simulink model "gm_HDLAWGNGenerator"  (R2021a)
settings: Solver=FixedStepDiscrete  StartTime=0.0  StopTime=StopTime  RelTol=1e-3
InitFcn:
  | whdlexamples.hdlawgn_init
undefined symbols (not defined in the file or in its folder): coefficientsSqrt1, coefficientsSqrt2, SamplingTime, seedsURNG1, seedsURNG2
libraries: hdlsllib x22, simulink x21, dspsrcs4 x1
(part 1 of 2)
settings Model: SimulationMode=accelerator  Creator=The MathWorks, Inc.  LastModifiedBy=huber
settings SolverCC: AlgebraicLoopSolver=TrustRegion
settings DataIOCC: ReturnWorkspaceOutputs=off
settings OptimizationCC: BlockReduction=off  ConditionallyExecuteInputs=off  DefaultParameterBehavior=Inlined
settings DebuggingCC: AlgebraicLoopMsg=error  InheritedTsInSrcMsg=none  SingleTaskRateTransMsg=error  IntegerOverflowMsg=none  ParameterPrecisionLossMsg=none  SFMachineParentedDataDiag=warning
settings HardwareCC: ProdBitPerPointer=32  ProdBitPerSizeT=32  ProdBitPerPtrDiffT=32  ProdLargestAtomicFloat=None  ProdIntDivRoundTo=Undefined  ProdEndianess=Unspecified  ProdWordSize=32  ProdHWDeviceType=ASIC/FPGA->ASIC/FPGA  TargetBitPerPointer=64  TargetBitPerSizeT=64  TargetBitPerPtrDiffT=64  TargetLongLongMode=on  TargetIntDivRoundTo=Zero  TargetEndianess=LittleEndian  TargetWordSize=64  TargetHWDeviceType=Custom Processor->MATLAB Host Computer  ProdEqTarget=off

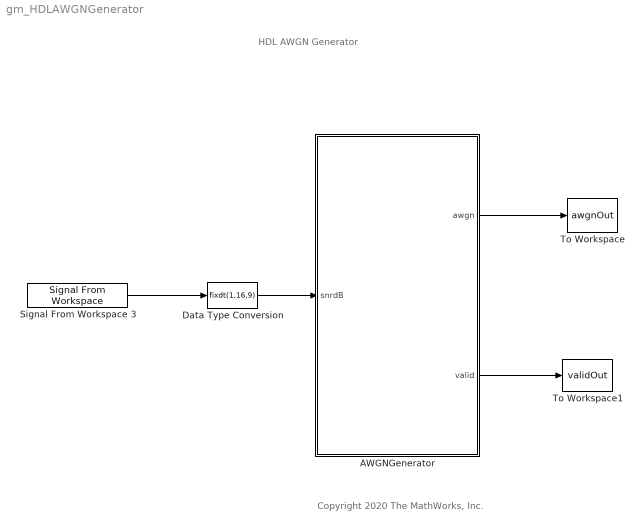
== system gm_HDLAWGNGenerator ==
  note: Copyright 2020 The MathWorks, Inc.
  note: HDL AWGN Generator
  AWGNGenerator : Subsystem
  Data Type Conversion : DataTypeConversion  OutDataTypeStr=fixdt(1,16,9)
  Signal From Workspace 3 : dspsrcs4/Signal From Workspace  X=snrdBSimInput  Ts=SamplingTime  nsamps=1  OutputAfterFinalValue=Setting to zero  ignoreOrWarnInputAndFrameLengths=on  OutputFrames=off
  To Workspace : ToWorkspace  VariableName=awgnOut  SampleTime=-1
      settings: Save2DSignal=2-D array (concatenate along first dimension)
  To Workspace1 : ToWorkspace  VariableName=validOut  SampleTime=-1
      settings: Save2DSignal=2-D array (concatenate along first dimension)
  wires:
  AWGNGenerator/2(valid) -> To Workspace1/1
  AWGNGenerator/1(awgn) -> To Workspace/1
  Data Type Conversion/1 -> AWGNGenerator/1(snrdB)
  Signal From Workspace 3/1 -> Data Type Conversion/1

== system gm_HDLAWGNGenerator/AWGNGenerator ==
  snrdB : Inport  OutDataTypeStr=fixdt(1, 16, 9)  PortDimensions=1  SampleTime=1e-06
  " dBtoLinearConverter" : Subsystem
  Data Type Conversion1 : DataTypeConversion  OutDataTypeStr=fixdt(1,16,9)
  Delay1 : Delay  DelayLength=10
  GaussianNoiseWithReqVar : Subsystem
  GaussianNoiseWithUnitVar : Subsystem
  awgn : Outport  SampleTime=1e-06
  valid : Outport  Port=2  SampleTime=1e-06
  wires:
  snrdB/1 -> Data Type Conversion1/1
  " dBtoLinearConverter"/1(noiseVar) -> Delay1/1
  Data Type Conversion1/1 -> " dBtoLinearConverter"/1(snrdB)
  Delay1/1 -> GaussianNoiseWithReqVar/1(noiseVar)
  GaussianNoiseWithReqVar/1(awgn) -> awgn/1
  GaussianNoiseWithReqVar/2(validOut) -> valid/1
  GaussianNoiseWithUnitVar/1(x0) -> GaussianNoiseWithReqVar/2(x0)
  GaussianNoiseWithUnitVar/2(x1) -> GaussianNoiseWithReqVar/3(x1)

== system gm_HDLAWGNGenerator/AWGNGenerator/ dBtoLinearConverter ==
  snrdB : Inport  OutDataTypeStr=fixdt(1, 16, 9)  PortDimensions=1  SampleTime=1e-06
  Add : Sum  AccumDataTypeStr=int16  OutDataTypeStr=int16  SampleTime=1e-06
  Constant : Constant  Value=201  OutDataTypeStr=int16  SampleTime=1e-06
  Delay1 : Delay  DelayLength=double(1)  InitialCondition=0  SampleTime=1e-06
  Gain : Gain  Gain="fi(0,1,16,11,\"hex\",\"5000\")"  ParamDataTypeStr=fixdt(1, 16, 11)  OutDataTypeStr=fixdt(1, 32, 20)  SampleTime=1e-06
  Gain_out_dtc : DataTypeConversion  OutDataTypeStr=int16  RndMeth=Round  SampleTime=1e-06
  sqrt(noisePow/2) : Lookup_n-D  NumberOfTableDimensions=1  BreakpointsForDimension1="fi(\"numerictype\",numerictype(1,16,0),\"fimath\",fimath(\"RoundingMethod\", \"Nearest\",\"OverflowAction\", \"Saturate\",\"ProductMode\",\"FullPrecision\",\"SumMode\",\"FullPrecision\"),\"Value\",\"[0 1 2 3 4 5 6 7 8 9 10 11 12 13 14 15 16 17 18 19 20 21 22 23 24 25 26 27 28 29 30 31 32 33 34 35 36 37 38 39 40 41 42 43 44 45 46 47 48 49 50 51 52 53 54 55 56 57 58 59 60 61 62 63 64 65 66 67 68 69 70 71 72 73 74 75 76 77 78 79 80 81 82 83 84 85 86 87 88 89 90 91 92 93 94 95 96 97 98 99 100 101 102 103 104 105 106 107 108 109 110 111 112 113 114 115 116 117 118 119 120 121 122 123 124 125 126 127 128 129 130 131 132 133 134 135 136 137 138 139 140 141 142 143 144 145 146 147 148 149 150 151 152 153 154 155 156 157 158 159 160 161 162 163 164 165 166 167 168 169 170 171 172 173 174 175 176 177 178 179 180 181 182 183 184 185 186 187 188 189 190 191 192 193 194 195 196 197 198 199 200 201 202 203 204 205 206 207 208 209 210 211 212 213 214 215 216 217 218 219 220 221 222 223 224 225 226 227 228 229 230 231 232 233 234 235 236 237 238 239 240 241 242 243 244 245 246 247 248 249 250 251 252 253 254 255 256 257 258 259 260 261 262 263 264 265 266 267 268 269 270 271 272 273 274 275 276 277 278 279 280 281 282 283 284 285 286 287 288 289 290 291 292 293 294 295 296 297 298 299 300 301 302 303 304 305 306 307 308 309 310 311 312 313 314 315 316 317 318 319 320 321 322 323 324 325 326 327 328 329 330 331 332 333 334 335 336 337 338 339 340 341 342 343 344 345 346 347 348 349 350 351 352 353 354 355 356 357 358 359 360 361 362 363 364 365 366 367 368 369 370 371 372 373 374 375 376 377 378 379 380 381 382 383 384 385 386 387 388 389 390 391 392 393 394 395 396 397 398 399 400 401 402 403 404 405 406 407 408 409 410 411 412 413 414 415 416 417 418 419 420 421 422 423 424 425 426 427 428 429 430 431 432 433 434 435 436 437 438 439 440 441 442 443 444 445 446 447 448 449 450 451 452 453 454 455 456 457 458 459 460 461 462 463 464 465 466 467 468 469 470 471 472 473 474 475 476 477 478 479 480 481 482 483 484 485 486 487 488 489 490 491 492 493 494 495 496 497 498 499 500 501 502 503 504 505 506 507 508 509 510 511]\")"  Table="reshape(fi(\"numerictype\",numerictype(0,22,18),\"fimath\",fimath(\"RoundingMethod\", \"Floor\",\"OverflowAction\", \"Wrap\",\"ProductMode\",\"FullPrecision\",\"SumMode\",\"FullPrecision\"),\"Value\",\"[0;7.07106781005859375;6.9901275634765625;6.9101104736328125;6.831012725830078125;6.752819061279296875;6.675518035888671875;6.5991058349609375;6.523563385009765625;6.44889068603515625;6.375072479248046875;6.302097320556640625;6.22995758056640625;6.158641815185546875;6.088146209716796875;6.01845550537109375;5.94956207275390625;5.881458282470703125;5.8141326904296875;5.74758148193359375;5.681789398193359375;5.616748809814453125;5.552455902099609375;5.488895416259765625;5.42606353759765625;5.36395263671875;5.30255126953125;5.241855621337890625;5.181850433349609375;5.12253570556640625;5.063899993896484375;5.005931854248046875;4.94863128662109375;4.8919830322265625;4.835987091064453125;4.780628204345703125;4.7259063720703125;4.67180633544921875;4.6183319091796875;4.565464019775390625;4.513202667236328125;4.461544036865234375;4.410472869873046875;4.3599853515625;4.310077667236328125;4.260738372802734375;4.21196746826171875;4.163753509521484375;4.116092681884765625;4.068973541259765625;4.022396087646484375;3.976352691650390625;3.930835723876953125;3.88584136962890625;3.841358184814453125;3.797389984130859375;3.7539215087890625;3.710948944091796875;3.668468475341796875;3.626476287841796875;3.584964752197265625;3.5439300537109375;3.503360748291015625;3.463260650634765625;3.423614501953125;3.384426116943359375;3.345684051513671875;3.3073883056640625;3.269527435302734375;3.2321014404296875;3.195102691650390625;3.15853118896484375;3.12237548828125;3.08663177490234375;3.051300048828125;3.0163726806640625;2.981845855712890625;2.947711944580078125;2.913970947265625;2.880615234375;2.8476409912109375;2.815044403076171875;2.782817840576171875;2.750965118408203125;2.71947479248046875;2.68834686279296875;2.65756988525390625;2.6271514892578125;2.597076416015625;2.567348480224609375;2.537960052490234375;2.5089111328125;2.480190277099609375;2.451801300048828125;2.423732757568359375;2.39598846435546875;2.368564605712890625;2.341449737548828125;2.314647674560546875;2.288150787353515625;2.261959075927734375;2.2360687255859375;2.21047210693359375;2.185169219970703125;2.16015625;2.13542938232421875;2.11098480224609375;2.086818695068359375;2.062931060791015625;2.039318084716796875;2.0159759521484375;1.99289703369140625;1.97008514404296875;1.94753265380859375;1.92523956298828125;1.903202056884765625;1.88141632080078125;1.8598785400390625;1.838588714599609375;1.81754302978515625;1.7967376708984375;1.776172637939453125;1.755840301513671875;1.73574066162109375;1.71587371826171875;1.696231842041015625;1.676815032958984375;1.657619476318359375;1.638645172119140625;1.6198883056640625;1.601345062255859375;1.58301544189453125;1.5648956298828125;1.5469818115234375;1.52927398681640625;1.511768341064453125;1.4944610595703125;1.47735595703125;1.460445404052734375;1.4437255859375;1.4272003173828125;1.410861968994140625;1.39471435546875;1.378749847412109375;1.362964630126953125;1.347362518310546875;1.331939697265625;1.3166961669921875;1.3016204833984375;1.286724090576171875;1.27199554443359375;1.257434844970703125;1.243038177490234375;1.228809356689453125;1.21474456787109375;1.200839996337890625;1.187091827392578125;1.173503875732421875;1.16007232666015625;1.146793365478515625;1.1336669921875;1.12068939208984375;1.107860565185546875;1.095180511474609375;1.0826416015625;1.070247650146484375;1.0579986572265625;1.045886993408203125;1.033916473388671875;1.0220794677734375;1.010379791259765625;0.998813629150390625;0.9873809814453125;0.976078033447265625;0.96490478515625;0.953861236572265625;0.942943572998046875;0.932147979736328125;0.921478271484375;0.910930633544921875;0.900501251220703125;0.890193939208984375;0.8800048828125;0.869930267333984375;0.859973907470703125;0.850128173828125;0.840396881103515625;0.830776214599609375;0.821269989013671875;0.81186676025390625;0.80257415771484375;0.79338836669921875;0.784305572509765625;0.775325775146484375;0.766452789306640625;0.757678985595703125;0.749004364013671875;0.7404327392578125;0.73195648193359375;0.723575592041015625 ...(+6252 chars)]\"), [1  512])"  InterpMethod=Flat  ExtrapMethod=Clip  DiagnosticForOutOfRangeInput=Error  SampleTime=1e-06  OutDataTypeStr=fixdt(0, 22, 18)  RndMeth=Simplest  InputSameDT=on
  noiseVar : Outport  SampleTime=1e-06
  wires:
  snrdB/1 -> Gain/1
  Add/1 -> Delay1/1
  Constant/1 -> Add/2
  Delay1/1 -> sqrt(noisePow/2)/1
  Gain_out_dtc/1 -> Add/1
  sqrt(noisePow/2)/1 -> noiseVar/1
  Gain/1 -> Gain_out_dtc/1

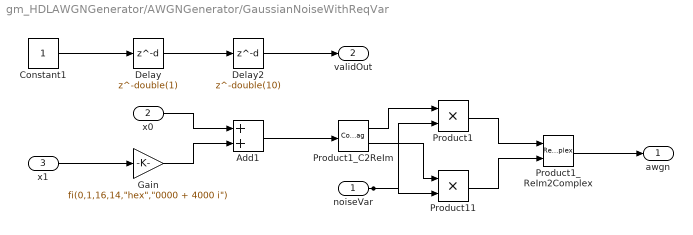
== system gm_HDLAWGNGenerator/AWGNGenerator/GaussianNoiseWithReqVar ==
  noiseVar : Inport  OutDataTypeStr=fixdt(0, 22, 18)  PortDimensions=1  SampleTime=1e-06
  x0 : Inport  Port=2  OutDataTypeStr=fixdt(1, 16, 11)  PortDimensions=1  SampleTime=1e-06
  x1 : Inport  Port=3  OutDataTypeStr=fixdt(1, 16, 11)  PortDimensions=1  SampleTime=1e-06
  Add1 : Sum  AccumDataTypeStr=fixdt(1, 33, 25)  OutDataTypeStr=fixdt(1, 16, 11)  SampleTime=1e-06
  Constant1 : Constant  OutDataTypeStr=boolean  SampleTime=1e-06
  Delay : Delay  DelayLength=double(1)  InitialCondition=0  SampleTime=1e-06
  Delay2 : Delay  DelayLength=double(10)  InitialCondition=0  SampleTime=1e-06
  Gain : Gain  Gain="fi(0,1,16,14,\"hex\",\"0000 + 4000 i\")"  ParamDataTypeStr=fixdt(1, 16, 14)  OutDataTypeStr=fixdt(1, 32, 25)  SampleTime=1e-06
  Product1 : Product  Inputs=**  OutDataTypeStr=fixdt(1, 38, 29)  SampleTime=1e-06
  Product11 : Product  Inputs=**  OutDataTypeStr=fixdt(1, 38, 29)  SampleTime=1e-06
  Product1_C2ReIm : ComplexToRealImag  SampleTime=1e-06
  Product1_ReIm2Complex : RealImagToComplex  SampleTime=1e-06
  awgn : Outport  SampleTime=1e-06
  validOut : Outport  Port=2  SampleTime=1e-06  VectorParamsAs1DForOutWhenUnconnected=off
  wires:
  noiseVar/1 -> Product11/2, Product1/2
  x0/1 -> Add1/1
  x1/1 -> Gain/1
  Add1/1 -> Product1_C2ReIm/1
  Constant1/1 -> Delay/1
  Delay/1 -> Delay2/1
  Delay2/1 -> validOut/1
  Gain/1 -> Add1/2
  Product1_ReIm2Complex/1 -> awgn/1
  Product1_C2ReIm/1 -> Product1/1
  Product1_C2ReIm/2 -> Product11/1
  Product1/1 -> Product1_ReIm2Complex/1
  Product11/1 -> Product1_ReIm2Complex/2

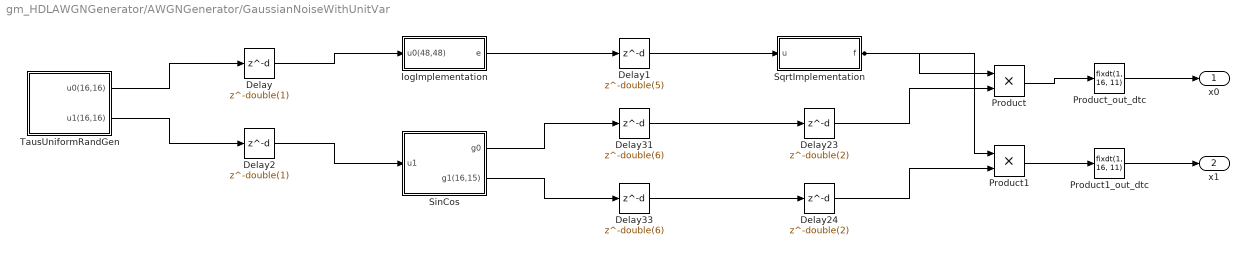
== system gm_HDLAWGNGenerator/AWGNGenerator/GaussianNoiseWithUnitVar ==
  Delay : Delay  DelayLength=double(1)  InitialCondition=0  SampleTime=1e-06
  Delay1 : Delay  DelayLength=double(5)  InitialCondition=0  SampleTime=1e-06
  Delay2 : Delay  DelayLength=double(1)  InitialCondition=0  SampleTime=1e-06
  Delay23 : Delay  DelayLength=double(2)  InitialCondition=0  SampleTime=1e-06
  Delay24 : Delay  DelayLength=double(2)  InitialCondition=0  SampleTime=1e-06
  Delay31 : Delay  DelayLength=double(6)  InitialCondition=0  SampleTime=1e-06
  Delay33 : Delay  DelayLength=double(6)  InitialCondition=0  SampleTime=1e-06
  Product : Product  Inputs=**  OutDataTypeStr=fixdt(1, 33, 28)  SampleTime=1e-06
  Product1 : Product  Inputs=**  OutDataTypeStr=fixdt(1, 33, 28)  SampleTime=1e-06
  Product1_out_dtc : DataTypeConversion  OutDataTypeStr=fixdt(1, 16, 11)  SampleTime=1e-06
  Product_out_dtc : DataTypeConversion  OutDataTypeStr=fixdt(1, 16, 11)  SampleTime=1e-06
  SinCos : Subsystem
  SqrtImplementation : Subsystem
  TausUniformRandGen : Subsystem
  logImplementation : Subsystem
  x0 : Outport  SampleTime=1e-06
  x1 : Outport  Port=2  SampleTime=1e-06
  wires:
  Delay/1 -> logImplementation/1(u0(48,48))
  Delay1/1 -> SqrtImplementation/1(u)
  Delay2/1 -> SinCos/1(u1)
  Delay23/1 -> Product/2
  Delay24/1 -> Product1/2
  Delay31/1 -> Delay23/1
  Delay33/1 -> Delay24/1
  Product_out_dtc/1 -> x0/1
  Product1_out_dtc/1 -> x1/1
  SinCos/1(g0) -> Delay31/1
  SinCos/2(g1(16,15)) -> Delay33/1
  SqrtImplementation/1(f) -> Product1/1, Product/1
  TausUniformRandGen/1(u0(16,16)) -> Delay/1
  TausUniformRandGen/2(u1(16,16)) -> Delay2/1
  logImplementation/1(e) -> Delay1/1
  Product/1 -> Product_out_dtc/1
  Product1/1 -> Product1_out_dtc/1

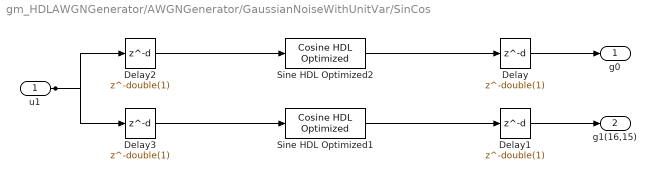
== system gm_HDLAWGNGenerator/AWGNGenerator/GaussianNoiseWithUnitVar/SinCos ==
  u1 : Inport  OutDataTypeStr=fixdt(0, 16, 16)  PortDimensions=1  SampleTime=1e-06
  Delay{,1..3} (4 alike) : Delay  DelayLength=double(1)  InitialCondition=0  SampleTime=1e-06
  Sine HDL Optimized1 : hdlsllib/Lookup Tables/Cosine HDL Optimized  OutputFormula=cos(2*pi*u)  NumDataPoints=1024  TableDataTypeStr=fixdt(0,15,15)  SimulateLUTROMDelay=off
      settings: SourceProductBaseCode=SL
  Sine HDL Optimized2 : hdlsllib/Lookup Tables/Cosine HDL Optimized  OutputFormula=sin(2*pi*u)  NumDataPoints=1024  TableDataTypeStr=fixdt(0,15,15)  SimulateLUTROMDelay=off
      settings: SourceProductBaseCode=SL
  g0 : Outport  SampleTime=1e-06
  g1(16,15) : Outport  Port=2  SampleTime=1e-06
  wires:
  u1/1 -> Delay2/1, Delay3/1
  Delay/1 -> g0/1
  Delay1/1 -> g1(16,15)/1
  Delay2/1 -> Sine HDL Optimized2/1
  Delay3/1 -> Sine HDL Optimized1/1
  Sine HDL Optimized1/1 -> Delay1/1
  Sine HDL Optimized2/1 -> Delay/1

== system gm_HDLAWGNGenerator/AWGNGenerator/GaussianNoiseWithUnitVar/SqrtImplementation ==
  u : Inport  OutDataTypeStr=fixdt(0, 31, 24)  PortDimensions=1  SampleTime=1e-06
  Constant : Constant  Value=0  OutDataTypeStr=fixdt(0,17,13)  SampleTime=-1
  Delay : Delay
  Delay1 : Delay
  SqrtEval : Subsystem
  Switch : Switch  Criteria=u2 ~= 0
  f : Outport  SampleTime=1e-06  VectorParamsAs1DForOutWhenUnconnected=off
  wires:
  u/1 -> Delay/1, SqrtEval/1(u)
  Constant/1 -> Delay1/1
  Delay/1 -> Switch/2
  Delay1/1 -> Switch/3
  SqrtEval/1(f) -> Switch/1
  Switch/1 -> f/1

== system gm_HDLAWGNGenerator/AWGNGenerator/GaussianNoiseWithUnitVar/TausUniformRandGen ==
  ConcatandExtract : Subsystem
  TausURNG1 : Subsystem
  TausURNG2 : Subsystem
  u0(16,16) : Outport  SampleTime=1e-06
  u1(16,16) : Outport  Port=2  SampleTime=1e-06
  wires:
  ConcatandExtract/1(u0(48,48)) -> u0(16,16)/1
  ConcatandExtract/2(u1(16,16)) -> u1(16,16)/1
  TausURNG1/1(a) -> ConcatandExtract/1(a)
  TausURNG2/1(b) -> ConcatandExtract/2(b)

== system gm_HDLAWGNGenerator/AWGNGenerator/GaussianNoiseWithUnitVar/logImplementation ==
  u0(48,48) : Inport  OutDataTypeStr=fixdt(0, 48, 48)  PortDimensions=1  SampleTime=1e-06
  Constant : Constant  Value=0  OutDataTypeStr=fixdt(0,16,9)  SampleTime=-1
  Delay : Delay  DelayLength=3
  Switch : Switch  Criteria=u2 ~= 0
  log : Subsystem
  e : Outport  SampleTime=1e-06
  wires:
  u0(48,48)/1 -> Delay/1, log/1(u0(48,48))
  Constant/1 -> Switch/3
  Delay/1 -> Switch/2
  Switch/1 -> e/1
  log/1(e) -> Switch/1

== system gm_HDLAWGNGenerator/AWGNGenerator/GaussianNoiseWithUnitVar/SqrtImplementation/SqrtEval ==
  u : Inport  OutDataTypeStr=fixdt(0, 31, 24)  PortDimensions=1  SampleTime=1e-06
  FunctionEvaluation : Subsystem
  RangeReconstruction : Subsystem
  RangeReduction : Subsystem
  f : Outport  SampleTime=1e-06
  wires:
  u/1 -> RangeReduction/1(u)
  FunctionEvaluation/1(y_f) -> RangeReconstruction/1(y_f)
  FunctionEvaluation/2(passOut) -> RangeReconstruction/2(pass)
  FunctionEvaluation/3(exp_fOut) -> RangeReconstruction/3(exp_f)
  RangeReconstruction/1(f) -> f/1
  RangeReduction/1(x_f) -> FunctionEvaluation/1(x_f)
  RangeReduction/2(pass) -> FunctionEvaluation/2(passIn)
  RangeReduction/3(exp_f) -> FunctionEvaluation/3(exp_fIn)

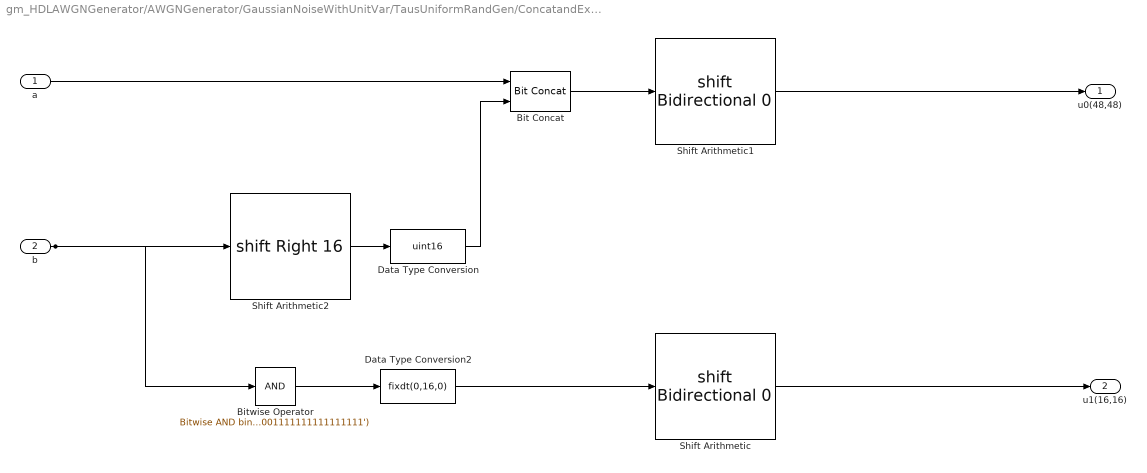
== system gm_HDLAWGNGenerator/AWGNGenerator/GaussianNoiseWithUnitVar/TausUniformRandGen/ConcatandExtract ==
  a : Inport  OutDataTypeStr=uint32  PortDimensions=1  SampleTime=1e-06
  b : Inport  Port=2  OutDataTypeStr=uint32  PortDimensions=1  SampleTime=1e-06
  Bit Concat : hdlsllib/Logic and Bit Operations/Bit Concat  numInputs=2
  Bitwise Operator : simulink/Logic and Bit Operations/Bitwise Operator  logicop=AND  UseBitMask=on  BitMask=bin2dec('00000000000000001111111111111111')  BitMaskRealWorld=Stored Integer
  Data Type Conversion : DataTypeConversion  OutDataTypeStr=uint16
  Data Type Conversion2 : DataTypeConversion  OutDataTypeStr=fixdt(0,16,0)
  Shift Arithmetic : ArithShift  BinPtShiftNumber=-16
  Shift Arithmetic1 : ArithShift  BinPtShiftNumber=-48
  Shift Arithmetic2 : ArithShift  BitShiftNumber=16  BitShiftDirection=Right
  u0(48,48) : Outport  SampleTime=1e-06
  u1(16,16) : Outport  Port=2  SampleTime=1e-06
  wires:
  a/1 -> Bit Concat/1
  b/1 -> Shift Arithmetic2/1, Bitwise Operator/1
  Bit Concat/1 -> Shift Arithmetic1/1
  Bitwise Operator/1 -> Data Type Conversion2/1
  Data Type Conversion/1 -> Bit Concat/2
  Data Type Conversion2/1 -> Shift Arithmetic/1
  Shift Arithmetic/1 -> u1(16,16)/1
  Shift Arithmetic1/1 -> u0(48,48)/1
  Shift Arithmetic2/1 -> Data Type Conversion/1

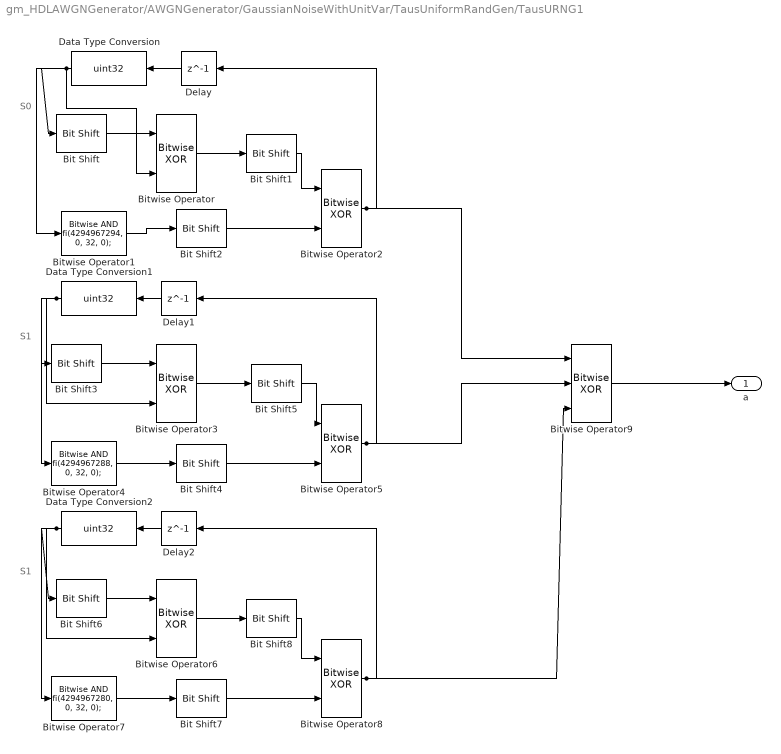
== system gm_HDLAWGNGenerator/AWGNGenerator/GaussianNoiseWithUnitVar/TausUniformRandGen/TausURNG1 ==
  note: S1
  note: S1
  note: S0
  Bit Shift : hdlsllib/Logic and Bit Operations/Bit Shift  mode=Shift Left Logical  N=13
  Bit Shift1 : hdlsllib/Logic and Bit Operations/Bit Shift  mode=Shift Right Logical  N=19
  Bit Shift2 : hdlsllib/Logic and Bit Operations/Bit Shift  mode=Shift Left Logical  N=12
  Bit Shift3 : hdlsllib/Logic and Bit Operations/Bit Shift  mode=Shift Left Logical  N=2
  Bit Shift4 : hdlsllib/Logic and Bit Operations/Bit Shift  mode=Shift Left Logical  N=4
  Bit Shift5 : hdlsllib/Logic and Bit Operations/Bit Shift  mode=Shift Right Logical  N=25
  Bit Shift6 : hdlsllib/Logic and Bit Operations/Bit Shift  mode=Shift Left Logical  N=3
  Bit Shift7 : hdlsllib/Logic and Bit Operations/Bit Shift  mode=Shift Left Logical  N=17
  Bit Shift8 : hdlsllib/Logic and Bit Operations/Bit Shift  mode=Shift Right Logical  N=11
  Bitwise Operator{,2..3,5..6,8} (6 alike) : simulink/Logic and Bit Operations/Bitwise Operator  logicop=XOR  UseBitMask=off  NumInputPorts=2  BitMask=bin2dec('11011001')  BitMaskRealWorld=Stored Integer
  Bitwise Operator1 : simulink/Logic and Bit Operations/Bitwise Operator  logicop=AND  UseBitMask=on  BitMask=fi(4294967294, 0, 32, 0);  BitMaskRealWorld=Stored Integer
  Bitwise Operator4 : simulink/Logic and Bit Operations/Bitwise Operator  logicop=AND  UseBitMask=on  BitMask=fi(4294967288, 0, 32, 0);  BitMaskRealWorld=Stored Integer
  Bitwise Operator7 : simulink/Logic and Bit Operations/Bitwise Operator  logicop=AND  UseBitMask=on  BitMask=fi(4294967280, 0, 32, 0);  BitMaskRealWorld=Stored Integer
  Bitwise Operator9 : simulink/Logic and Bit Operations/Bitwise Operator  logicop=XOR  UseBitMask=off  NumInputPorts=3  BitMask=bin2dec('11011001')  BitMaskRealWorld=Stored Integer
  Data Type Conversion : DataTypeConversion  OutDataTypeStr=uint32
  Data Type Conversion1 : DataTypeConversion  OutDataTypeStr=uint32
  Data Type Conversion2 : DataTypeConversion  OutDataTypeStr=uint32
  Delay : Delay  DelayLength=1  InitialCondition=seedsURNG1(1)
  Delay1 : Delay  DelayLength=1  InitialCondition=seedsURNG1(2)
  Delay2 : Delay  DelayLength=1  InitialCondition=seedsURNG1(3)
  a : Outport  SampleTime=1e-06
  wires:
  Bit Shift/1 -> Bitwise Operator/1
  Bit Shift1/1 -> Bitwise Operator2/1
  Bit Shift2/1 -> Bitwise Operator2/2
  Bit Shift3/1 -> Bitwise Operator3/1
  Bit Shift4/1 -> Bitwise Operator5/2
  Bit Shift5/1 -> Bitwise Operator5/1
  Bit Shift6/1 -> Bitwise Operator6/1
  Bit Shift7/1 -> Bitwise Operator8/2
  Bit Shift8/1 -> Bitwise Operator8/1
  Bitwise Operator/1 -> Bit Shift1/1
  Bitwise Operator1/1 -> Bit Shift2/1
  Bitwise Operator2/1 -> Bitwise Operator9/1, Delay/1
  Bitwise Operator3/1 -> Bit Shift5/1
  Bitwise Operator4/1 -> Bit Shift4/1
  Bitwise Operator5/1 -> Bitwise Operator9/2, Delay1/1
  Bitwise Operator6/1 -> Bit Shift8/1
  Bitwise Operator7/1 -> Bit Shift7/1
  Bitwise Operator8/1 -> Bitwise Operator9/3, Delay2/1
  Bitwise Operator9/1 -> a/1
  Data Type Conversion/1 -> Bitwise Operator1/1, Bitwise Operator/2, Bit Shift/1
  Data Type Conversion1/1 -> Bitwise Operator4/1, Bitwise Operator3/2, Bit Shift3/1
  Data Type Conversion2/1 -> Bitwise Operator7/1, Bitwise Operator6/2, Bit Shift6/1
  Delay/1 -> Data Type Conversion/1
  Delay1/1 -> Data Type Conversion1/1
  Delay2/1 -> Data Type Conversion2/1

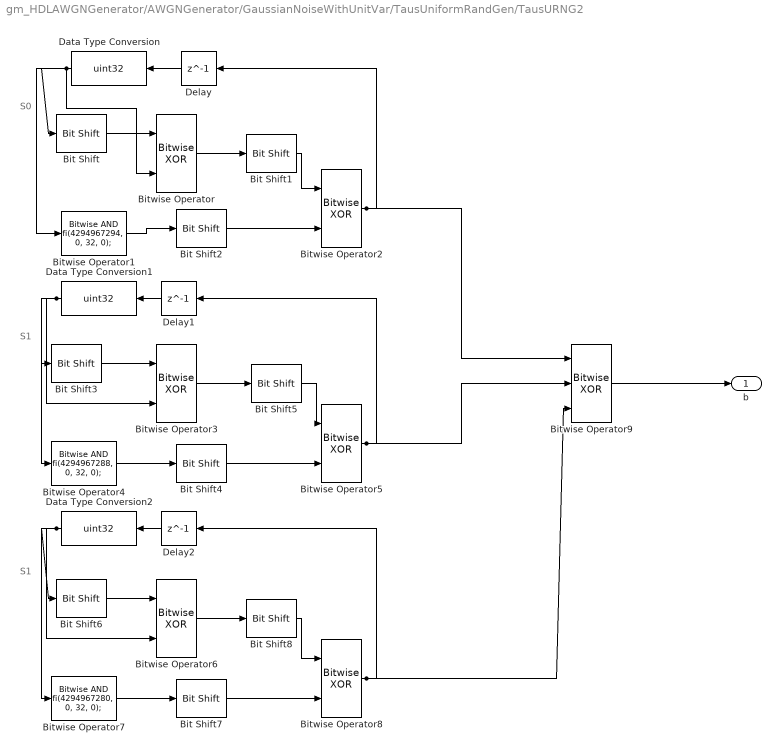
== system gm_HDLAWGNGenerator/AWGNGenerator/GaussianNoiseWithUnitVar/TausUniformRandGen/TausURNG2 ==
  note: S1
  note: S1
  note: S0
  Bit Shift : hdlsllib/Logic and Bit Operations/Bit Shift  mode=Shift Left Logical  N=13
  Bit Shift1 : hdlsllib/Logic and Bit Operations/Bit Shift  mode=Shift Right Logical  N=19
  Bit Shift2 : hdlsllib/Logic and Bit Operations/Bit Shift  mode=Shift Left Logical  N=12
  Bit Shift3 : hdlsllib/Logic and Bit Operations/Bit Shift  mode=Shift Left Logical  N=2
  Bit Shift4 : hdlsllib/Logic and Bit Operations/Bit Shift  mode=Shift Left Logical  N=4
  Bit Shift5 : hdlsllib/Logic and Bit Operations/Bit Shift  mode=Shift Right Logical  N=25
  Bit Shift6 : hdlsllib/Logic and Bit Operations/Bit Shift  mode=Shift Left Logical  N=3
  Bit Shift7 : hdlsllib/Logic and Bit Operations/Bit Shift  mode=Shift Left Logical  N=17
  Bit Shift8 : hdlsllib/Logic and Bit Operations/Bit Shift  mode=Shift Right Logical  N=11
  Bitwise Operator{,2..3,5..6,8} (6 alike) : simulink/Logic and Bit Operations/Bitwise Operator  logicop=XOR  UseBitMask=off  NumInputPorts=2  BitMask=bin2dec('11011001')  BitMaskRealWorld=Stored Integer
  Bitwise Operator1 : simulink/Logic and Bit Operations/Bitwise Operator  logicop=AND  UseBitMask=on  BitMask=fi(4294967294, 0, 32, 0);  BitMaskRealWorld=Stored Integer
  Bitwise Operator4 : simulink/Logic and Bit Operations/Bitwise Operator  logicop=AND  UseBitMask=on  BitMask=fi(4294967288, 0, 32, 0);  BitMaskRealWorld=Stored Integer
  Bitwise Operator7 : simulink/Logic and Bit Operations/Bitwise Operator  logicop=AND  UseBitMask=on  BitMask=fi(4294967280, 0, 32, 0);  BitMaskRealWorld=Stored Integer
  Bitwise Operator9 : simulink/Logic and Bit Operations/Bitwise Operator  logicop=XOR  UseBitMask=off  NumInputPorts=3  BitMask=bin2dec('11011001')  BitMaskRealWorld=Stored Integer
  Data Type Conversion : DataTypeConversion  OutDataTypeStr=uint32
  Data Type Conversion1 : DataTypeConversion  OutDataTypeStr=uint32
  Data Type Conversion2 : DataTypeConversion  OutDataTypeStr=uint32
  Delay : Delay  DelayLength=1  InitialCondition=seedsURNG2(1)
  Delay1 : Delay  DelayLength=1  InitialCondition=seedsURNG2(2)
  Delay2 : Delay  DelayLength=1  InitialCondition=seedsURNG2(3)
  b : Outport  SampleTime=1e-06
  wires:
  Bit Shift/1 -> Bitwise Operator/1
  Bit Shift1/1 -> Bitwise Operator2/1
  Bit Shift2/1 -> Bitwise Operator2/2
  Bit Shift3/1 -> Bitwise Operator3/1
  Bit Shift4/1 -> Bitwise Operator5/2
  Bit Shift5/1 -> Bitwise Operator5/1
  Bit Shift6/1 -> Bitwise Operator6/1
  Bit Shift7/1 -> Bitwise Operator8/2
  Bit Shift8/1 -> Bitwise Operator8/1
  Bitwise Operator/1 -> Bit Shift1/1
  Bitwise Operator1/1 -> Bit Shift2/1
  Bitwise Operator2/1 -> Bitwise Operator9/1, Delay/1
  Bitwise Operator3/1 -> Bit Shift5/1
  Bitwise Operator4/1 -> Bit Shift4/1
  Bitwise Operator5/1 -> Bitwise Operator9/2, Delay1/1
  Bitwise Operator6/1 -> Bit Shift8/1
  Bitwise Operator7/1 -> Bit Shift7/1
  Bitwise Operator8/1 -> Bitwise Operator9/3, Delay2/1
  Bitwise Operator9/1 -> b/1
  Data Type Conversion/1 -> Bitwise Operator1/1, Bitwise Operator/2, Bit Shift/1
  Data Type Conversion1/1 -> Bitwise Operator4/1, Bitwise Operator3/2, Bit Shift3/1
  Data Type Conversion2/1 -> Bitwise Operator7/1, Bitwise Operator6/2, Bit Shift6/1
  Delay/1 -> Data Type Conversion/1
  Delay1/1 -> Data Type Conversion1/1
  Delay2/1 -> Data Type Conversion2/1

== system gm_HDLAWGNGenerator/AWGNGenerator/GaussianNoiseWithUnitVar/logImplementation/log ==
  u0(48,48) : Inport  OutDataTypeStr=fixdt(0, 48, 48)  PortDimensions=1  SampleTime=1e-06
  FunctionEvaluation : Subsystem
  RangeReconstruction : Subsystem
  RangeReduction : Subsystem
  e : Outport  SampleTime=1e-06  VectorParamsAs1DForOutWhenUnconnected=off
  wires:
  u0(48,48)/1 -> RangeReduction/1(x)
  FunctionEvaluation/1(y_e) -> RangeReconstruction/1(y_e)
  FunctionEvaluation/2(exp_eOut) -> RangeReconstruction/2(exp_e)
  RangeReconstruction/1(e) -> e/1
  RangeReduction/1(x_e) -> FunctionEvaluation/1(x_e)
  RangeReduction/2(exp_e) -> FunctionEvaluation/2(exp_eIn)

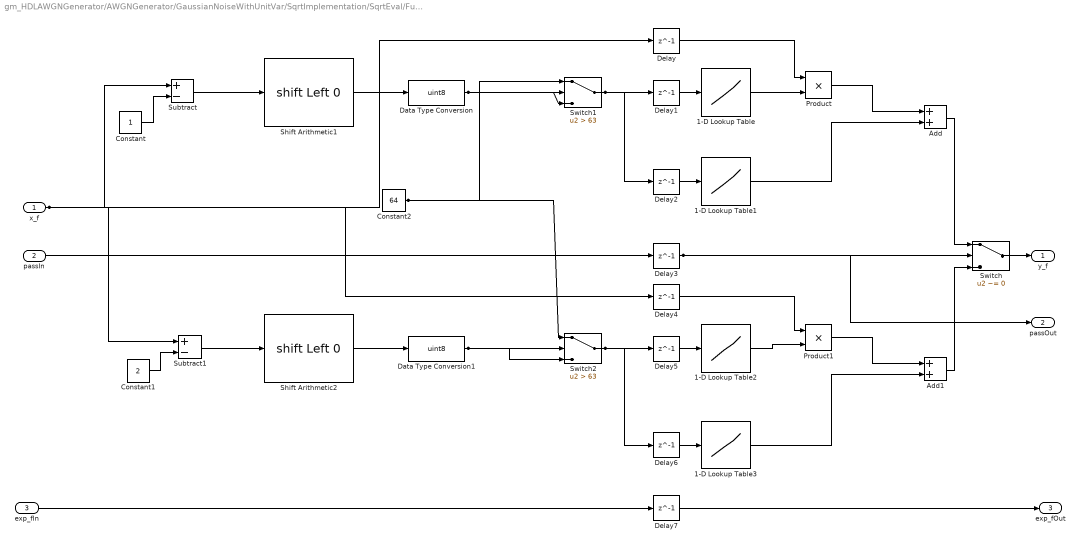
== system gm_HDLAWGNGenerator/AWGNGenerator/GaussianNoiseWithUnitVar/SqrtImplementation/SqrtEval/FunctionEvaluation ==
  x_f : Inport  OutDataTypeStr=fixdt(0, 31, 24)  PortDimensions=1  SampleTime=1e-06
  passIn : Inport  Port=2  OutDataTypeStr=fixdt(1, 9, 0)  PortDimensions=1  SampleTime=1e-06
  exp_fIn : Inport  Port=3  OutDataTypeStr=int8  PortDimensions=1  SampleTime=1e-06
  1-D Lookup Table : Lookup_n-D  NumberOfTableDimensions=1  LookupTableObject=''  BreakpointsForDimension1=[0:64]  BreakpointsForDimension1FirstPoint=10  BreakpointsForDimension2FirstPoint=10  BreakpointsForDimension1Spacing=12  BreakpointsForDimension2Spacing=12  IndexSearchMethod=Evenly spaced points  Table=[coefficientsSqrt1(:,1)' 0]  InterpMethod=Flat  DiagnosticForOutOfRangeInput=Error  InternalRulePriority=Speed  OutDataTypeStr=fixdt(1,13,12)  RndMeth=Simplest  InputSameDT=on
  1-D Lookup Table1 : Lookup_n-D  NumberOfTableDimensions=1  LookupTableObject=''  BreakpointsForDimension1=0:64  BreakpointsForDimension1FirstPoint=10  BreakpointsForDimension2FirstPoint=10  BreakpointsForDimension1Spacing=12  BreakpointsForDimension2Spacing=12  IndexSearchMethod=Evenly spaced points  Table=[coefficientsSqrt1(:,2)' 0]  InterpMethod=Flat  DiagnosticForOutOfRangeInput=Error  InternalRulePriority=Speed  OutDataTypeStr=fixdt(1,21,20)  RndMeth=Simplest  InputSameDT=on
  1-D Lookup Table2 : Lookup_n-D  NumberOfTableDimensions=1  LookupTableObject=''  BreakpointsForDimension1=0:64  BreakpointsForDimension1FirstPoint=10  BreakpointsForDimension2FirstPoint=10  BreakpointsForDimension1Spacing=12  BreakpointsForDimension2Spacing=12  IndexSearchMethod=Evenly spaced points  Table=[coefficientsSqrt2(:,1)' 0]  InterpMethod=Flat  DiagnosticForOutOfRangeInput=Error  InternalRulePriority=Speed  OutDataTypeStr=fixdt(1,13,12)  RndMeth=Simplest  InputSameDT=on
  1-D Lookup Table3 : Lookup_n-D  NumberOfTableDimensions=1  LookupTableObject=''  BreakpointsForDimension1=0:64  BreakpointsForDimension1FirstPoint=10  BreakpointsForDimension2FirstPoint=10  BreakpointsForDimension1Spacing=12  BreakpointsForDimension2Spacing=12  IndexSearchMethod=Evenly spaced points  Table=[coefficientsSqrt2(:,2)' 0]  InterpMethod=Flat  DiagnosticForOutOfRangeInput=Error  InternalRulePriority=Speed  OutDataTypeStr=fixdt(1,21,20)  RndMeth=Simplest  InputSameDT=on
  Add : Sum  OutDataTypeStr=fixdt(0,17,13)
  Add1 : Sum  AccumDataTypeStr=fixdt(0,17,13)
  Constant : Constant  OutDataTypeStr=uint8  SampleTime=-1
  Constant1 : Constant  Value=2  OutDataTypeStr=uint8  SampleTime=-1
  Constant2 : Constant  Value=64  OutDataTypeStr=uint8  SampleTime=-1
  Data Type Conversion : DataTypeConversion  OutDataTypeStr=uint8
  Data Type Conversion1 : DataTypeConversion  OutDataTypeStr=uint8
  Delay{,1..7} (8 alike) : Delay  DelayLength=1
  Product : Product
  Product1 : Product
  Shift Arithmetic1 : ArithShift  BinPtShiftNumber=6  BitShiftDirection=Left
  Shift Arithmetic2 : ArithShift  BinPtShiftNumber=5  BitShiftDirection=Left
  Subtract : Sum  Inputs=+-
  Subtract1 : Sum  Inputs=+-  AccumDataTypeStr=fixdt(0,31,24)
  Switch : Switch  Criteria=u2 ~= 0
  Switch1 : Switch  Criteria=u2 > Threshold  Threshold=63
  Switch2 : Switch  Criteria=u2 > Threshold  Threshold=63  OutDataTypeStr=int8
  y_f : Outport  SampleTime=1e-06
  passOut : Outport  Port=2  SampleTime=1e-06
  exp_fOut : Outport  Port=3  SampleTime=1e-06
  wires:
  x_f/1 -> Subtract1/1, Subtract/1, Delay4/1, Delay/1
  passIn/1 -> Delay3/1
  exp_fIn/1 -> Delay7/1
  1-D Lookup Table/1 -> Product/2
  1-D Lookup Table1/1 -> Add/2
  1-D Lookup Table2/1 -> Product1/2
  1-D Lookup Table3/1 -> Add1/2
  Add/1 -> Switch/1
  Add1/1 -> Switch/3
  Constant/1 -> Subtract/2
  Constant1/1 -> Subtract1/2
  Constant2/1 -> Switch2/1, Switch1/1
  Data Type Conversion/1 -> Switch1/3, Switch1/2
  Data Type Conversion1/1 -> Switch2/3, Switch2/2
  Delay/1 -> Product/1
  Delay1/1 -> 1-D Lookup Table/1
  Delay2/1 -> 1-D Lookup Table1/1
  Delay3/1 -> Switch/2, passOut/1
  Delay4/1 -> Product1/1
  Delay5/1 -> 1-D Lookup Table2/1
  Delay6/1 -> 1-D Lookup Table3/1
  Delay7/1 -> exp_fOut/1
  Product/1 -> Add/1
  Product1/1 -> Add1/1
  Shift Arithmetic1/1 -> Data Type Conversion/1
  Shift Arithmetic2/1 -> Data Type Conversion1/1
  Subtract/1 -> Shift Arithmetic1/1
  Subtract1/1 -> Shift Arithmetic2/1
  Switch/1 -> y_f/1
  Switch1/1 -> Delay2/1, Delay1/1
  Switch2/1 -> Delay6/1, Delay5/1

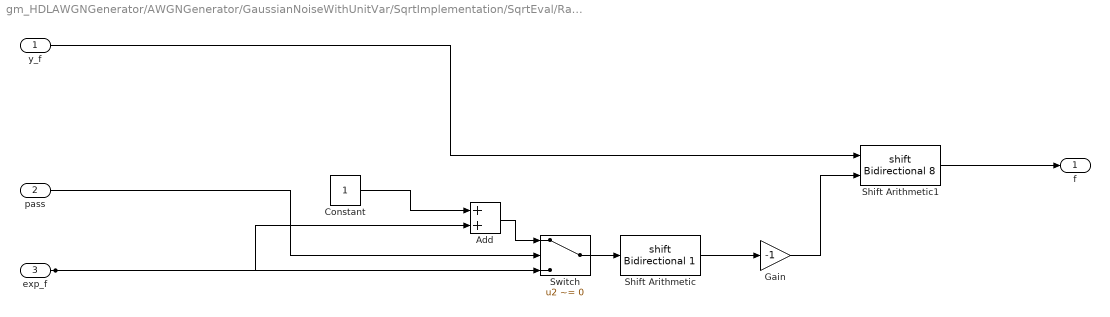
== system gm_HDLAWGNGenerator/AWGNGenerator/GaussianNoiseWithUnitVar/SqrtImplementation/SqrtEval/RangeReconstruction ==
  y_f : Inport  OutDataTypeStr=fixdt(0, 17, 13)  PortDimensions=1  SampleTime=1e-06
  pass : Inport  Port=2  OutDataTypeStr=fixdt(1, 9, 0)  PortDimensions=1  SampleTime=1e-06
  exp_f : Inport  Port=3  OutDataTypeStr=int8  PortDimensions=1  SampleTime=1e-06
  Add : Sum  AccumDataTypeStr=int8
  Constant : Constant  OutDataTypeStr=int8  SampleTime=-1
  Gain : Gain  Gain=-1  OutDataTypeStr=int8
  Shift Arithmetic : ArithShift  BitShiftNumber=1
  Shift Arithmetic1 : ArithShift  BitShiftNumberSource=Input port  BitShiftNumber=8
      settings: InputPortMap=u0,p1
  Switch : Switch  Criteria=u2 ~= 0
  f : Outport  SampleTime=1e-06
  wires:
  y_f/1 -> Shift Arithmetic1/1
  pass/1 -> Switch/2
  exp_f/1 -> Switch/3, Add/2
  Add/1 -> Switch/1
  Constant/1 -> Add/1
  Gain/1 -> Shift Arithmetic1/2
  Shift Arithmetic/1 -> Gain/1
  Shift Arithmetic1/1 -> f/1
  Switch/1 -> Shift Arithmetic/1

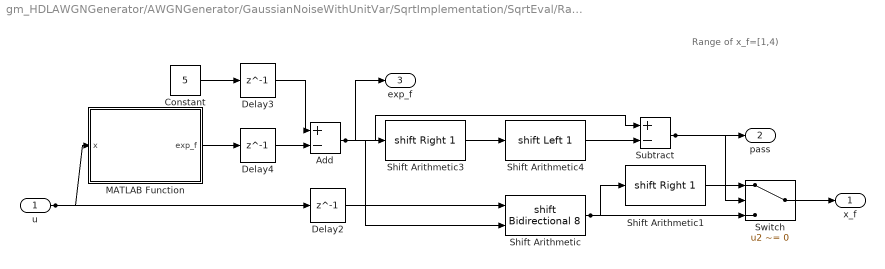
== system gm_HDLAWGNGenerator/AWGNGenerator/GaussianNoiseWithUnitVar/SqrtImplementation/SqrtEval/RangeReduction ==
  note: Range of x_f=[1,4)
  u : Inport  OutDataTypeStr=fixdt(0, 31, 24)  PortDimensions=1  SampleTime=1e-06
  Add : Sum  Inputs=+-  OutDataTypeStr=int8
  Constant : Constant  Value=5  OutDataTypeStr=uint8  SampleTime=-1
  Delay2 : Delay  DelayLength=1
  Delay3 : Delay  DelayLength=1
  Delay4 : Delay  DelayLength=1
  MATLAB Function : Subsystem
  Shift Arithmetic : ArithShift  BitShiftNumberSource=Input port  BitShiftNumber=8
      settings: InputPortMap=u0,p1
  Shift Arithmetic1 : ArithShift  BitShiftNumber=1  BitShiftDirection=Right
  Shift Arithmetic3 : ArithShift  BitShiftNumber=1  BitShiftDirection=Right
  Shift Arithmetic4 : ArithShift  BitShiftNumber=1  BitShiftDirection=Left
  Subtract : Sum  Inputs=+-
  Switch : Switch  Criteria=u2 ~= 0
  x_f : Outport  SampleTime=1e-06
  pass : Outport  Port=2  SampleTime=1e-06
  exp_f : Outport  Port=3  SampleTime=1e-06  VectorParamsAs1DForOutWhenUnconnected=off
  wires:
  u/1 -> Delay2/1, MATLAB Function/1(x)
  Add/1 -> Subtract/1, Shift Arithmetic3/1, Shift Arithmetic/2, exp_f/1
  Constant/1 -> Delay3/1
  Delay2/1 -> Shift Arithmetic/1
  Delay3/1 -> Add/1
  Delay4/1 -> Add/2
  MATLAB Function/1(exp_f) -> Delay4/1
  Shift Arithmetic/1 -> Switch/3, Shift Arithmetic1/1
  Shift Arithmetic1/1 -> Switch/1
  Shift Arithmetic3/1 -> Shift Arithmetic4/1
  Shift Arithmetic4/1 -> Subtract/2
  Subtract/1 -> Switch/2, pass/1
  Switch/1 -> x_f/1
